simulink model "MotorControl_Bldc"  (R2022a)
settings: Solver=ode4  StartTime=0.0  StopTime=1  FixedStep=Ts/cnt_pTs  RelTol=1e-3
values from neighbouring files (symbols this model uses):
  cnt_pTs = 1000    [motorpara.m]
  Fc = 1/Ts    (= 10000)    [motorpara.m]
  Ki_id = Rs*Fc    (= 4500)    [motorpara.m]
  Ki_iq = Rs*Fc    (= 4500)    [motorpara.m]
  Ki_v = 0.93    [motorpara.m]
  Kp_id = Ls*Fc    (= 4.2)    [motorpara.m]
  Kp_iq = Ls*Fc    (= 4.2)    [motorpara.m]
  Kp_v = 0.05    [motorpara.m]
  Ls = 0.00042    [motorpara.m]
  P = 2    [motorpara.m]
  Rs = 0.45    [motorpara.m]
  SMO_Kslide = 10    [motorpara.m]
  Ts = 1/10000    (= 0.0001)    [motorpara.m]
  V = 12    [motorpara.m]
undefined symbols (not defined in the file or in its folder): DiscIntNeverNeededParam, sigbuilder_block
libraries: nesl_utility x83, fl_lib x67, ee_lib x49, simulink x13, slpidlib x3, mcbplantlib x2, autolibpmsmexterior x1
(part 4 of 4)

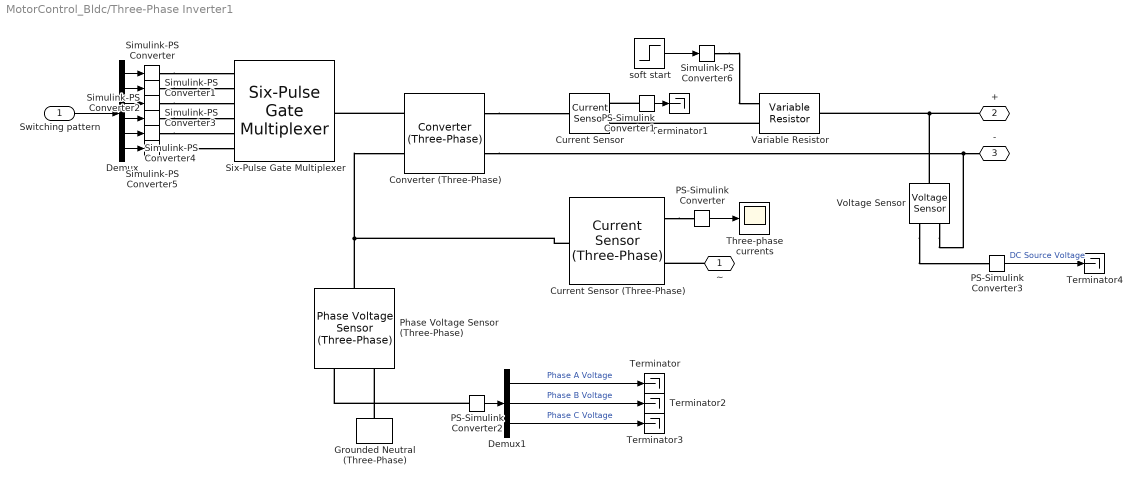
== system MotorControl_Bldc/Three-Phase Inverter1 ==
  Switching pattern : Inport
  Converter (Three-Phase) : ee_lib/Semiconductors & Converters/Converters/Converter (Three-Phase)  port_option=ee.enum.threePhasePort.composite  device_type=ee.enum.converters.switchingdevice.ideal  Vf=0.8 V  Ron=0.001 Ohm  Rds=0.001 Ohm  Goff=0.001 1/Ohm  Vgt=1 V  Vgt_off=-1 V  Ih=1 A  Vth=0.5 V  diode_param=ee.enum.converters.protectiondiode.nodynamics  diode_Vf=0.8 V  diode_Ron=0.001 Ohm  diode_Goff=1e-5 1/Ohm  diode_C=50 nF  diode_iRM=-235 A  diode_iF=300 A  diode_idot=-50 A/us  diode_trr_param=ee.enum.converters.diodetrr.trr_factor  diode_trr_factor=3  diode_trr=15 us  diode_Qrr=1500 s*uA  snubber_type=ee.enum.converters.snubber.exclude  Cs=1e-7 F  Rs=0.1 Ohm
      settings: SourceProductBaseCode=PS
  Current Sensor : fl_lib/Electrical/Electrical Sensors/Current Sensor
  Current Sensor (Three-Phase) : ee_lib/Sensors & Transducers/Current Sensor (Three-Phase)
  Demux : Demux  Outputs=6
  Demux1 : Demux  Outputs=3
  Grounded Neutral (Three-Phase) : ee_lib/Connectors & References/Grounded Neutral (Three-Phase)
      settings: SourceProductBaseCode=PS
  PS-Simulink Converter : nesl_utility/PS-Simulink Converter  PhysicalDomain=network_engine_domain  SubClassName=ps_output  LeftPortType=input  RightPortType=output  PseudoPeriodic=off  Frequencies=[]  VectorFormat=1-D array  Unit=1  AffineConversion=off
  PS-Simulink Converter1 : nesl_utility/PS-Simulink Converter  PhysicalDomain=network_engine_domain  SubClassName=ps_output  LeftPortType=input  RightPortType=output  PseudoPeriodic=off  Frequencies=[]  VectorFormat=1-D array  Unit=inherit  AffineConversion=off
  PS-Simulink Converter2 : nesl_utility/PS-Simulink Converter  PhysicalDomain=network_engine_domain  SubClassName=ps_output  LeftPortType=input  RightPortType=output  PseudoPeriodic=off  Frequencies=[]  VectorFormat=1-D array  Unit=inherit  AffineConversion=off
  PS-Simulink Converter3 : nesl_utility/PS-Simulink Converter  PhysicalDomain=network_engine_domain  SubClassName=ps_output  LeftPortType=input  RightPortType=output  PseudoPeriodic=off  Frequencies=[]  VectorFormat=1-D array  Unit=inherit  AffineConversion=off
  Phase Voltage Sensor (Three-Phase) : ee_lib/Sensors & Transducers/Phase Voltage Sensor (Three-Phase)
      settings: SourceProductBaseCode=PS
  Simulink-PS Converter{,1..6} (7 alike) : nesl_utility/Simulink-PS Converter  PhysicalDomain=network_engine_domain  SubClassName=ps_input  LeftPortType=input  RightPortType=output  PseudoPeriodic=off  Frequencies=[]  NoiseDistribution=none  NoiseParameters=[]  Unit=1  AffineConversion=off  FilteringAndDerivatives=provide  SimscapeFilterOrder=1  InputFilterTimeConstant=0.001  UdotUserProvided=0
  Six-Pulse Gate Multiplexer : ee_lib/Semiconductors & Converters/Converters/Six-Pulse Gate Multiplexer  port_option=ee.enum.controlport.ps
      settings: SourceProductBaseCode=PS
  Terminator{,1..4} (5 alike) : Terminator
  Three-phase currents : Scope
  Variable Resistor : fl_lib/Electrical/Electrical Elements/Variable Resistor  Rmin=0 Ohm  i_specify=off  i_priority=None  i=0 A  i_nominal_specify=off  i_nominal_unit=A  i_nominal_value=1  v_specify=off  v_priority=None  v=0 V  v_nominal_specify=off  v_nominal_unit=V  v_nominal_value=1
  Voltage Sensor : fl_lib/Electrical/Electrical Sensors/Voltage Sensor
  soft start : Step  Time=4  Before=0.5  After=1e-3  SampleTime=Ts
  ~ : PMIOPort  Side=Right
  + : PMIOPort  Port=2  Side=Left
  - : PMIOPort  Port=3  Side=Left
  wires:
  PS-Simulink Converter/1 -> Three-phase currents/1
  Switching pattern/1 -> Demux/1
  Demux/1 -> Simulink-PS Converter/1
  Demux/2 -> Simulink-PS Converter1/1
  Demux/3 -> Simulink-PS Converter2/1
  Demux/4 -> Simulink-PS Converter3/1
  Demux/5 -> Simulink-PS Converter4/1
  Demux/6 -> Simulink-PS Converter5/1
  PS-Simulink Converter2/1 -> Demux1/1
  soft start/1 -> Simulink-PS Converter6/1
  PS-Simulink Converter1/1 -> Terminator1/1
  Demux1/1 -> Terminator/1  "Phase A Voltage"
  Demux1/2 -> Terminator2/1  "Phase B Voltage"
  Demux1/3 -> Terminator3/1  "Phase C Voltage"
  PS-Simulink Converter3/1 -> Terminator4/1  "DC Source Voltage"
  connections:
  Current Sensor (Three-Phase)/RConn1 -- PS-Simulink Converter/LConn1
  Simulink-PS Converter/RConn1 -- Six-Pulse Gate Multiplexer/LConn1
  Simulink-PS Converter1/RConn1 -- Six-Pulse Gate Multiplexer/LConn2
  Simulink-PS Converter2/RConn1 -- Six-Pulse Gate Multiplexer/LConn3
  Simulink-PS Converter3/RConn1 -- Six-Pulse Gate Multiplexer/LConn4
  Simulink-PS Converter4/RConn1 -- Six-Pulse Gate Multiplexer/LConn5
  Simulink-PS Converter5/RConn1 -- Six-Pulse Gate Multiplexer/LConn6
  Converter (Three-Phase)/LConn1 -- Six-Pulse Gate Multiplexer/RConn1
  Converter (Three-Phase)/RConn1 -- Current Sensor/LConn1
  Converter (Three-Phase)/RConn2 -- Voltage Sensor/RConn2 -- -/RConn1
  Current Sensor (Three-Phase)/LConn1 -- Converter (Three-Phase)/LConn2 -- Phase Voltage Sensor (Three-Phase)/LConn1
  ~/RConn1 -- Current Sensor (Three-Phase)/RConn2
  Grounded Neutral (Three-Phase)/LConn1 -- Phase Voltage Sensor (Three-Phase)/RConn2
  PS-Simulink Converter2/LConn1 -- Phase Voltage Sensor (Three-Phase)/RConn1
  PS-Simulink Converter1/LConn1 -- Current Sensor/RConn1
  Variable Resistor/LConn2 -- Current Sensor/RConn2
  +/RConn1 -- Voltage Sensor/LConn1 -- Variable Resistor/RConn1
  Simulink-PS Converter6/RConn1 -- Variable Resistor/LConn1
  Voltage Sensor/RConn1 -- PS-Simulink Converter3/LConn1

== system MotorControl_Bldc/Tload1 ==
  Simulink-PS Converter4 : nesl_utility/Simulink-PS Converter  PhysicalDomain=network_engine_domain  SubClassName=ps_input  LeftPortType=input  RightPortType=output  PseudoPeriodic=off  Frequencies=[]  NoiseDistribution=none  NoiseParameters=[]  Unit=N*m  AffineConversion=off  FilteringAndDerivatives=zero  SimscapeFilterOrder=1  InputFilterTimeConstant=0.001  UdotUserProvided=1
      settings: SourceProductBaseCode=SS,PW,VE
  Step : Step  Time=0.9  After=-2  SampleTime=0
  Tload : PMIOPort  Side=Right
  wires:
  Step/1 -> Simulink-PS Converter4/1
  connections:
  Simulink-PS Converter4/RConn1 -- Tload/RConn1

== system MotorControl_Bldc/Tload3 ==
  Simulink-PS Converter4 : nesl_utility/Simulink-PS Converter  PhysicalDomain=network_engine_domain  SubClassName=ps_input  LeftPortType=input  RightPortType=output  PseudoPeriodic=off  Frequencies=[]  NoiseDistribution=none  NoiseParameters=[]  Unit=N*m  AffineConversion=off  FilteringAndDerivatives=zero  SimscapeFilterOrder=1  InputFilterTimeConstant=0.001  UdotUserProvided=1
      settings: SourceProductBaseCode=SS,PW,VE
  Step : Step  Time=0.9  After=-2  SampleTime=0
  Tload : PMIOPort  Side=Right
  wires:
  Step/1 -> Simulink-PS Converter4/1
  connections:
  Simulink-PS Converter4/RConn1 -- Tload/RConn1

== system MotorControl_Bldc/clark ==
  PhI : Inport
  Add : Sum
  Demux : Demux  Outputs=3
  Gain : Gain  Gain=2
  Gain1 : Gain  Gain=1/sqrt(3)
  Scope : Scope
  Iα : Outport
  Iβ : Outport  Port=2
  wires:
  PhI/1 -> Demux/1
  Demux/1 -> Add/1, Iα/1
  Demux/2 -> Gain/1
  Gain/1 -> Add/2
  Add/1 -> Gain1/1
  Gain1/1 -> Iβ/1
  Demux/3 -> Scope/1

== system MotorControl_Bldc/ref_ratio ==
  alpha : Inport
  lead : Inport  Port=2
  leg : Inport  Port=3
  Add7 : Sum
  Cos : Trigonometry  Operator=cos
  Sin : Trigonometry
  Sqrt : Sqrt
  ap : Product
  bp : Product
  mcos : Product
  msin : Product
  module : Outport
  wires:
  ap/1 -> msin/2, msin/1
  Add7/1 -> Sqrt/1
  Cos/1 -> bp/1
  mcos/1 -> Add7/2
  Sin/1 -> ap/2
  alpha/1 -> Cos/1, Sin/1
  bp/1 -> mcos/1, mcos/2
  Sqrt/1 -> module/1
  msin/1 -> Add7/1
  lead/1 -> bp/2
  leg/1 -> ap/1

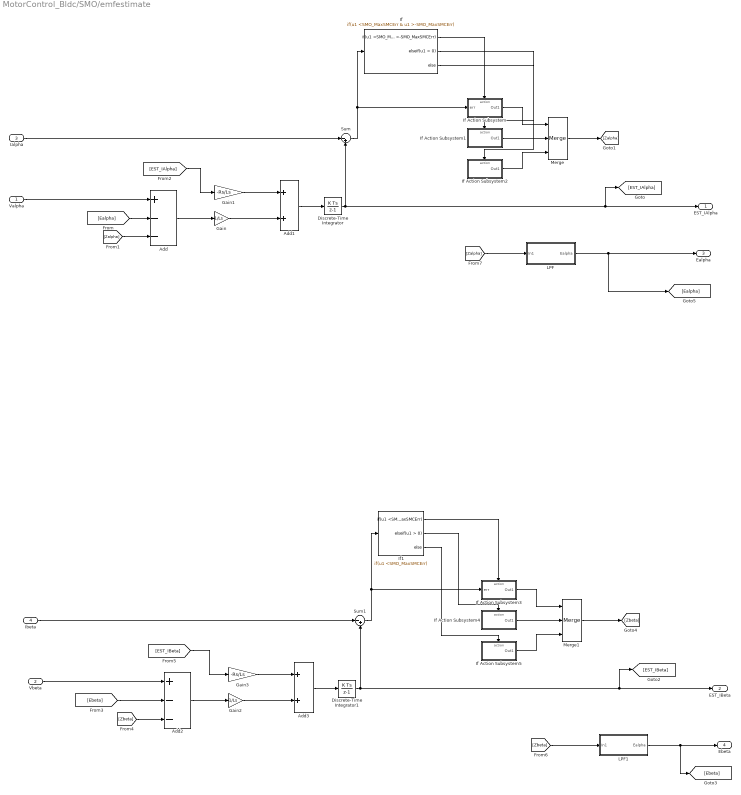
== system MotorControl_Bldc/SMO/emfestimate ==
  Valpha : Inport
  Vbeta : Inport  Port=2
  Ialpha : Inport  Port=3
  Ibeta : Inport  Port=4
  Add : Sum  Inputs=+--
  Add1 : Sum
  Add2 : Sum  Inputs=+--
  Add3 : Sum
  Discrete-Time Integrator : DiscreteIntegrator  SampleTime=Ts  ICPrevOutput=DiscIntNeverNeededParam  ICPrevScaledInput=DiscIntNeverNeededParam
  Discrete-Time Integrator1 : DiscreteIntegrator  SampleTime=Ts  ICPrevOutput=DiscIntNeverNeededParam  ICPrevScaledInput=DiscIntNeverNeededParam
  Gain : Gain  Gain=1/Ls
  Gain1 : Gain  Gain=-Rs/Ls
  Gain2 : Gain  Gain=1/Ls
  Gain3 : Gain  Gain=-Rs/Ls
  If : If  IfExpression=u1 <SMO_MaxSMCErr & u1 >-SMO_MaxSMCErr  ElseIfExpressions=u1 > 0
  If Action Subsystem : Subsystem  TreatAsAtomicUnit=on
  If Action Subsystem1 : Subsystem  TreatAsAtomicUnit=on
  If Action Subsystem2 : Subsystem  TreatAsAtomicUnit=on
  If Action Subsystem3 : Subsystem  TreatAsAtomicUnit=on
  If Action Subsystem4 : Subsystem  TreatAsAtomicUnit=on
  If Action Subsystem5 : Subsystem  TreatAsAtomicUnit=on
  If1 : If  IfExpression=u1 <SMO_MaxSMCErr  ElseIfExpressions=u1 > 0
  LPF : Subsystem
  LPF1 : Subsystem
  Merge : Merge  Inputs=3
  Merge1 : Merge  Inputs=3
  Sum : Sum  Inputs=|-+
  Sum1 : Sum  Inputs=|-+
  EST_IAlpha : Outport
  EST_IBeta : Outport  Port=2
  Ealpha : Outport  Port=3
  Ebeta : Outport  Port=4
  wires:
  Valpha/1 -> Add/1
  Add/1 -> Gain/1
  [Ealpha] -> Add/2
  [Zalpha] -> Add/3
  Gain/1 -> Add1/2
  Gain1/1 -> Add1/1
  [EST_IAlpha] -> Gain1/1
  Add1/1 -> Discrete-Time Integrator/1
  Discrete-Time Integrator/1 -> [EST_IAlpha], EST_IAlpha/1, Sum/2
  Ialpha/1 -> Sum/1
  Sum/1 -> If/1, If Action Subsystem/1(err)
  If/1 -> If Action Subsystem/Action
  If/2 -> If Action Subsystem1/Action
  If/3 -> If Action Subsystem2/Action
  If Action Subsystem1/1(Out1) -> Merge/2
  If Action Subsystem/1(Out1) -> Merge/1
  If Action Subsystem2/1(Out1) -> Merge/3
  Merge/1 -> [Zalpha]
  Add3/1 -> Discrete-Time Integrator1/1
  [Zbeta] -> Add2/3
  If Action Subsystem5/1(Out1) -> Merge1/3
  Gain2/1 -> Add3/2
  Merge1/1 -> [Zbeta]
  If Action Subsystem3/1(Out1) -> Merge1/1
  If Action Subsystem4/1(Out1) -> Merge1/2
  Vbeta/1 -> Add2/1
  [Ebeta] -> Add2/2
  Ibeta/1 -> Sum1/1
  Sum1/1 -> If1/1, If Action Subsystem3/1(err)
  If1/3 -> If Action Subsystem5/Action
  If1/1 -> If Action Subsystem3/Action
  Gain3/1 -> Add3/1
  Discrete-Time Integrator1/1 -> EST_IBeta/1, [EST_IBeta], Sum1/2
  [EST_IBeta] -> Gain3/1
  If1/2 -> If Action Subsystem4/Action
  Add2/1 -> Gain2/1
  LPF/1(Ealpha) -> [Ealpha], Ealpha/1
  [Zalpha] -> LPF/1(In1)
  LPF1/1(Ealpha) -> [Ebeta], Ebeta/1
  [Zbeta] -> LPF1/1(In1)

== system MotorControl_Bldc/SMO/vmeasure ==
  last : Inport
  this : Inport  Port=2
  Add : Sum  Inputs=-+
  Constant : Constant  Value=Ts
  Divide : Product  Inputs=*/
  Gain : Gain  Gain=30/pi
  If : If  IfExpression=u1 > 4.7  ElseIfExpressions=u1<-4.7
  If Action Subsystem : Subsystem  TreatAsAtomicUnit=on
  If Action Subsystem1 : Subsystem  TreatAsAtomicUnit=on
  If Action Subsystem2 : Subsystem  TreatAsAtomicUnit=on
  Merge : Merge  Inputs=3
  Saturation : Saturate  UpperLimit=5000  LowerLimit=-5000
  Out1 : Outport
  wires:
  last/1 -> If Action Subsystem/2(last), If Action Subsystem1/2(last), Add/1
  this/1 -> If Action Subsystem1/1(this), If Action Subsystem/1(this), Add/2
  Add/1 -> If/1, If Action Subsystem2/1(In1)
  If/1 -> If Action Subsystem/Action
  If/2 -> If Action Subsystem1/Action
  If/3 -> If Action Subsystem2/Action
  If Action Subsystem2/1(Out1) -> Merge/2
  If Action Subsystem/1(Out1) -> Merge/1
  Merge/1 -> Divide/1
  Divide/1 -> Gain/1
  Constant/1 -> Divide/2
  If Action Subsystem1/1(Out1) -> Merge/3
  Gain/1 -> Saturation/1
  Saturation/1 -> Out1/1

== system MotorControl_Bldc/SVPWM/Sector ==
  Vα : Inport
  Vβ : Inport  Port=2
  Add : Sum  Inputs=+-
  Add1 : Sum  Inputs=--
  Add2 : Sum  Inputs=+++
  Constant : Constant
  Constant1 : Constant  Value=0
  Gain : Gain  Gain=sqrt(3)
  Gain1 : Gain  Gain=4
  Gain2 : Gain  Gain=2
  Gain3 : Gain
  Switch : Switch  Criteria=u2 > Threshold  SaturateOnIntegerOverflow=off  InputSameDT=off
  Switch1 : Switch  Criteria=u2 > Threshold  SaturateOnIntegerOverflow=off  InputSameDT=off
  Switch2 : Switch  Criteria=u2 > Threshold  SaturateOnIntegerOverflow=off  InputSameDT=off
  N : Outport
  wires:
  Vα/1 -> Gain/1
  Gain/1 -> Add1/1, Add/1
  Vβ/1 -> Add1/2, Switch/2, Add/2
  Add/1 -> Switch1/2
  Add1/1 -> Switch2/2
  Constant1/1 -> Switch/3, Switch1/3, Switch2/3
  Constant/1 -> Switch2/1, Switch1/1, Switch/1
  Switch/1 -> Gain3/1
  Switch1/1 -> Gain2/1
  Switch2/1 -> Gain1/1
  Gain3/1 -> Add2/1
  Gain2/1 -> Add2/2
  Gain1/1 -> Add2/3
  Add2/1 -> N/1

== system MotorControl_Bldc/SVPWM/Subsystem ==
  N : Inport
  T1 : Inport  Port=2
  T2 : Inport  Port=3
  TS : Inport  Port=4
  Add : Sum  Inputs=--+
  Gain : Gain  Gain=0.5
  Gain1 : Gain  Gain=0.5
  Gain2 : Gain  Gain=1/4
  Index Vector : MultiPortSwitch  Inputs=6  DiagnosticForDefault=None  SaturateOnIntegerOverflow=off  InputSameDT=off
  Index Vector1 : MultiPortSwitch  Inputs=6  DiagnosticForDefault=None  SaturateOnIntegerOverflow=off  InputSameDT=off
  Index Vector2 : MultiPortSwitch  Inputs=6  DiagnosticForDefault=None  SaturateOnIntegerOverflow=off  InputSameDT=off
  mid1 : Sum
  mid2 : Sum
  Ta : Outport
  Tb : Outport  Port=2
  Tc : Outport  Port=3
  wires:
  T1/1 -> Add/2, Gain1/1
  T2/1 -> Add/1, Gain/1
  TS/1 -> Add/3
  Add/1 -> Gain2/1
  Gain/1 -> mid1/1
  Gain1/1 -> mid2/1
  mid2/1 -> Index Vector2/6, Index Vector2/3, Index Vector1/5, Index Vector1/4, Index Vector/7, Index Vector/2, mid1/2
  Gain2/1 -> Index Vector1/6, Index Vector1/2, Index Vector/4, Index Vector/3, mid2/2, Index Vector2/7, Index Vector2/5
  N/1 -> Index Vector2/1, Index Vector1/1, Index Vector/1
  mid1/1 -> Index Vector/6, Index Vector/5, Index Vector1/7, Index Vector2/4, Index Vector2/2, Index Vector1/3
  Index Vector/1 -> Ta/1
  Index Vector1/1 -> Tb/1
  Index Vector2/1 -> Tc/1

== system MotorControl_Bldc/SVPWM/T1T2 ==
  N : Inport
  X : Inport  Port=2
  Y : Inport  Port=3
  Z : Inport  Port=4
  Gain : Gain  Gain=-1
  Gain1 : Gain  Gain=-1
  Gain2 : Gain  Gain=-1
  Index Vector : MultiPortSwitch  Inputs=6  DiagnosticForDefault=None  SaturateOnIntegerOverflow=off  InputSameDT=off
  Index Vector1 : MultiPortSwitch  Inputs=6  DiagnosticForDefault=None  SaturateOnIntegerOverflow=off  InputSameDT=off
  T1 : Outport
  T2 : Outport  Port=2
  wires:
  X/1 -> Gain/1, Index Vector/6, Index Vector1/4
  Index Vector1/1 -> T2/1
  N/1 -> Index Vector1/1, Index Vector/1
  Y/1 -> Gain1/1, Index Vector/3, Index Vector1/2
  Z/1 -> Gain2/1, Index Vector1/5, Index Vector/2
  Gain/1 -> Index Vector1/3, Index Vector/5
  Gain2/1 -> Index Vector1/7, Index Vector/4
  Gain1/1 -> Index Vector/7, Index Vector1/6
  Index Vector/1 -> T1/1

== system MotorControl_Bldc/SVPWM/XYZ ==
  Vα : Inport
  Vβ : Inport  Port=2
  Vbus : Inport  Port=3
  TS : Inport  Port=4
  Add : Sum  Inputs=+-
  Add1 : Sum  Inputs=--
  Constant : Constant  Value=sqrt(3)
  Divide : Product  Inputs=**/
  Gain : Gain  Gain=sqrt(3)
  Gain1 : Gain  Gain=-0.5
  Gain2 : Gain  Gain=-0.5
  Product : Product
  Product1 : Product
  Product2 : Product
  X : Outport
  Y : Outport  Port=2
  Z : Outport  Port=3
  wires:
  Vα/1 -> Gain/1
  Gain/1 -> Add/1, Add1/1
  Vβ/1 -> Add1/2, Product/1, Add/2
  Add1/1 -> Gain1/1
  Add/1 -> Gain2/1
  Constant/1 -> Divide/1
  Vbus/1 -> Divide/3
  TS/1 -> Divide/2
  Gain1/1 -> Product1/1
  Divide/1 -> Product2/2, Product/2, Product1/2
  Product2/1 -> Z/1
  Product1/1 -> Y/1
  Product/1 -> X/1
  Gain2/1 -> Product2/1

== system MotorControl_Bldc/SVPWM1/Sector ==
  Vα : Inport
  Vβ : Inport  Port=2
  Add : Sum  Inputs=+-
  Add1 : Sum  Inputs=--
  Add2 : Sum  Inputs=+++
  Constant : Constant
  Constant1 : Constant  Value=0
  Gain : Gain  Gain=sqrt(3)
  Gain1 : Gain  Gain=4
  Gain2 : Gain  Gain=2
  Gain3 : Gain
  Switch : Switch  Criteria=u2 > Threshold  SaturateOnIntegerOverflow=off  InputSameDT=off
  Switch1 : Switch  Criteria=u2 > Threshold  SaturateOnIntegerOverflow=off  InputSameDT=off
  Switch2 : Switch  Criteria=u2 > Threshold  SaturateOnIntegerOverflow=off  InputSameDT=off
  N : Outport
  wires:
  Vα/1 -> Gain/1
  Gain/1 -> Add1/1, Add/1
  Vβ/1 -> Add1/2, Switch/2, Add/2
  Add/1 -> Switch1/2
  Add1/1 -> Switch2/2
  Constant1/1 -> Switch/3, Switch1/3, Switch2/3
  Constant/1 -> Switch2/1, Switch1/1, Switch/1
  Switch/1 -> Gain3/1
  Switch1/1 -> Gain2/1
  Switch2/1 -> Gain1/1
  Gain3/1 -> Add2/1
  Gain2/1 -> Add2/2
  Gain1/1 -> Add2/3
  Add2/1 -> N/1

== system MotorControl_Bldc/SVPWM1/Subsystem ==
  N : Inport
  T1 : Inport  Port=2
  T2 : Inport  Port=3
  TS : Inport  Port=4
  Add : Sum  Inputs=--+
  Gain : Gain  Gain=0.5
  Gain1 : Gain  Gain=0.5
  Gain2 : Gain  Gain=1/4
  Index Vector : MultiPortSwitch  Inputs=6  DiagnosticForDefault=None  SaturateOnIntegerOverflow=off  InputSameDT=off
  Index Vector1 : MultiPortSwitch  Inputs=6  DiagnosticForDefault=None  SaturateOnIntegerOverflow=off  InputSameDT=off
  Index Vector2 : MultiPortSwitch  Inputs=6  DiagnosticForDefault=None  SaturateOnIntegerOverflow=off  InputSameDT=off
  mid1 : Sum
  mid2 : Sum
  Ta : Outport
  Tb : Outport  Port=2
  Tc : Outport  Port=3
  wires:
  T1/1 -> Add/2, Gain1/1
  T2/1 -> Add/1, Gain/1
  TS/1 -> Add/3
  Add/1 -> Gain2/1
  Gain/1 -> mid1/1
  Gain1/1 -> mid2/1
  mid2/1 -> Index Vector2/6, Index Vector2/3, Index Vector1/5, Index Vector1/4, Index Vector/7, Index Vector/2, mid1/2
  Gain2/1 -> Index Vector1/6, Index Vector1/2, Index Vector/4, Index Vector/3, mid2/2, Index Vector2/7, Index Vector2/5
  N/1 -> Index Vector2/1, Index Vector1/1, Index Vector/1
  mid1/1 -> Index Vector/6, Index Vector/5, Index Vector1/7, Index Vector2/4, Index Vector2/2, Index Vector1/3
  Index Vector/1 -> Ta/1
  Index Vector1/1 -> Tb/1
  Index Vector2/1 -> Tc/1

== system MotorControl_Bldc/SVPWM1/T1T2 ==
  N : Inport
  X : Inport  Port=2
  Y : Inport  Port=3
  Z : Inport  Port=4
  Gain : Gain  Gain=-1
  Gain1 : Gain  Gain=-1
  Gain2 : Gain  Gain=-1
  Index Vector : MultiPortSwitch  Inputs=6  DiagnosticForDefault=None  SaturateOnIntegerOverflow=off  InputSameDT=off
  Index Vector1 : MultiPortSwitch  Inputs=6  DiagnosticForDefault=None  SaturateOnIntegerOverflow=off  InputSameDT=off
  T1 : Outport
  T2 : Outport  Port=2
  wires:
  X/1 -> Gain/1, Index Vector/6, Index Vector1/4
  Index Vector1/1 -> T2/1
  N/1 -> Index Vector1/1, Index Vector/1
  Y/1 -> Gain1/1, Index Vector/3, Index Vector1/2
  Z/1 -> Gain2/1, Index Vector1/5, Index Vector/2
  Gain/1 -> Index Vector1/3, Index Vector/5
  Gain2/1 -> Index Vector1/7, Index Vector/4
  Gain1/1 -> Index Vector/7, Index Vector1/6
  Index Vector/1 -> T1/1

== system MotorControl_Bldc/SVPWM1/XYZ ==
  Vα : Inport
  Vβ : Inport  Port=2
  Vbus : Inport  Port=3
  TS : Inport  Port=4
  Add : Sum  Inputs=+-
  Add1 : Sum  Inputs=--
  Constant : Constant  Value=sqrt(3)
  Divide : Product  Inputs=**/
  Gain : Gain  Gain=sqrt(3)
  Gain1 : Gain  Gain=-0.5
  Gain2 : Gain  Gain=-0.5
  Product : Product
  Product1 : Product
  Product2 : Product
  X : Outport
  Y : Outport  Port=2
  Z : Outport  Port=3
  wires:
  Vα/1 -> Gain/1
  Gain/1 -> Add/1, Add1/1
  Vβ/1 -> Add1/2, Product/1, Add/2
  Add1/1 -> Gain1/1
  Add/1 -> Gain2/1
  Constant/1 -> Divide/1
  Vbus/1 -> Divide/3
  TS/1 -> Divide/2
  Gain1/1 -> Product1/1
  Divide/1 -> Product2/2, Product/2, Product1/2
  Product2/1 -> Z/1
  Product1/1 -> Y/1
  Product/1 -> X/1
  Gain2/1 -> Product2/1

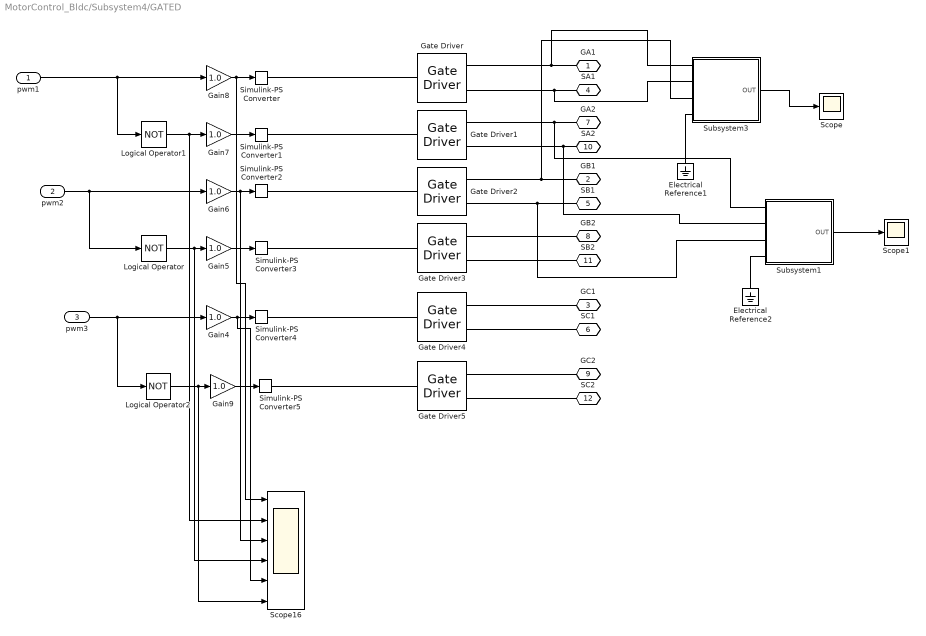
== system MotorControl_Bldc/Subsystem4/GATED ==
  pwm1 : Inport
  pwm2 : Inport  Port=2
  pwm3 : Inport  Port=3
  Electrical Reference1 : fl_lib/Electrical/Electrical Elements/Electrical Reference
      settings: SourceProductBaseCode=PW,SS,VE
  Electrical Reference2 : fl_lib/Electrical/Electrical Elements/Electrical Reference
      settings: SourceProductBaseCode=PW,SS,VE
  Gain{4..9} (6 alike) : Gain  Gain=1.0  OutDataTypeStr=double
  Gate Driver{,1..5} (6 alike) : ee_lib/Semiconductors & Converters/Gate Driver  uHighValue=0.7  uLowValue=0.3  vHigh=15 V  vLow=0 V  tHigh=50 ns  tLow=50 ns  parameterization=1  rHigh=2 Ohm  rLow=2 Ohm  tRise=20 ns  tFall=20 ns  cLoad=10 nF  enable_faults=0  t_fault=1 s  fault_type=1  ZonTime_specify=off  ZonTime_priority=None  ZonTime=0 s  ZoffTime_specify=off  ZoffTime_priority=None  ZoffTime=0 s  uHigh=2.0 V  uLow=0.8 V
      settings: SourceProductBaseCode=PS  InternalSimscapePortConfiguration="{\"Bottom\":[],\"Left\":[{\"id\":\"u\",\"label\":\"u\",\"type\":\"input\"}],\"Right\":[{\"id\":\"G\",\"label\":\"G\",\"type\":\"foundation.electrical.electrical\"},{\"id\":\"S\",\"label\":\"S\",\"type\":\"foundation.electrical.electrical\"}],\"Top\":[]}"
  Logical Operator : Logic  Operator=NOT  AllPortsSameDT=off  OutDataTypeStr=boolean
  Logical Operator1 : Logic  Operator=NOT  AllPortsSameDT=off  OutDataTypeStr=boolean
  Logical Operator2 : Logic  Operator=NOT  AllPortsSameDT=off  OutDataTypeStr=boolean
  Scope : Scope
  Scope1 : Scope
  Scope16 : Scope  NumInputPorts=6
  Simulink-PS Converter{,1..5} (6 alike) : nesl_utility/Simulink-PS Converter  PhysicalDomain=network_engine_domain  SubClassName=ps_input  LeftPortType=input  RightPortType=output  PseudoPeriodic=off  Frequencies=[]  NoiseDistribution=none  NoiseParameters=[]  Unit=1  AffineConversion=off  FilteringAndDerivatives=provide  SimscapeFilterOrder=1  InputFilterTimeConstant=0.001  UdotUserProvided=0
      settings: SourceProductBaseCode=SS,PW,VE
  Subsystem1 : Subsystem
  Subsystem3 : Subsystem
  GA1 : PMIOPort  Side=Right
  GB1 : PMIOPort  Port=2  Side=Right
  GC1 : PMIOPort  Port=3  Side=Right
  SA1 : PMIOPort  Port=4  Side=Right
  SB1 : PMIOPort  Port=5  Side=Right
  SC1 : PMIOPort  Port=6  Side=Right
  GA2 : PMIOPort  Port=7  Side=Right
  GB2 : PMIOPort  Port=8  Side=Right
  GC2 : PMIOPort  Port=9  Side=Right
  SA2 : PMIOPort  Port=10  Side=Right
  SB2 : PMIOPort  Port=11  Side=Right
  SC2 : PMIOPort  Port=12  Side=Right
  wires:
  Logical Operator2/1 -> Scope16/6, Gain9/1
  pwm2/1 -> Gain6/1, Logical Operator/1
  Gain5/1 -> Simulink-PS Converter3/1
  pwm3/1 -> Gain4/1, Logical Operator2/1
  Gain4/1 -> Scope16/5, Simulink-PS Converter4/1
  pwm1/1 -> Gain8/1, Logical Operator1/1
  Logical Operator/1 -> Scope16/4, Gain5/1
  Gain6/1 -> Scope16/3, Simulink-PS Converter2/1
  Gain7/1 -> Simulink-PS Converter1/1
  Gain8/1 -> Scope16/1, Simulink-PS Converter/1
  Gain9/1 -> Simulink-PS Converter5/1
  Logical Operator1/1 -> Scope16/2, Gain7/1
  Subsystem3/1(OUT) -> Scope/1
  Subsystem1/1(OUT) -> Scope1/1
  connections:
  Gate Driver3/LConn1 -- Simulink-PS Converter3/RConn1
  Gate Driver5/LConn1 -- Simulink-PS Converter5/RConn1
  Gate Driver/LConn1 -- Simulink-PS Converter/RConn1
  Gate Driver1/LConn1 -- Simulink-PS Converter1/RConn1
  Simulink-PS Converter2/RConn1 -- Gate Driver2/LConn1
  Gate Driver4/LConn1 -- Simulink-PS Converter4/RConn1
  GA1/RConn1 -- Subsystem3/LConn1 -- Gate Driver/RConn1
  SA1/RConn1 -- Subsystem3/LConn2 -- Gate Driver/RConn2
  GA2/RConn1 -- Subsystem1/LConn1 -- Gate Driver1/RConn1
  SA2/RConn1 -- Subsystem1/LConn2 -- Gate Driver1/RConn2
  GB1/RConn1 -- Subsystem3/LConn3 -- Gate Driver2/RConn1
  SB1/RConn1 -- Subsystem1/LConn3 -- Gate Driver2/RConn2
  GB2/RConn1 -- Gate Driver3/RConn1
  SB2/RConn1 -- Gate Driver3/RConn2
  GC1/RConn1 -- Gate Driver4/RConn1
  SC1/RConn1 -- Gate Driver4/RConn2
  GC2/RConn1 -- Gate Driver5/RConn1
  SC2/RConn1 -- Gate Driver5/RConn2
  Electrical Reference1/LConn1 -- Subsystem3/LConn4
  Electrical Reference2/LConn1 -- Subsystem1/LConn4

== system MotorControl_Bldc/Subsystem4/Subsystem3 ==
  Mux4 : Mux  Inputs=3
  PS-Simulink Converter : nesl_utility/PS-Simulink Converter  PhysicalDomain=network_engine_domain  SubClassName=ps_output  LeftPortType=input  RightPortType=output  PseudoPeriodic=off  Frequencies=[]  VectorFormat=inherit  Unit=inherit  AffineConversion=off
      settings: SourceProductBaseCode=SS,PW,VE
  PS-Simulink Converter1 : nesl_utility/PS-Simulink Converter  PhysicalDomain=network_engine_domain  SubClassName=ps_output  LeftPortType=input  RightPortType=output  PseudoPeriodic=off  Frequencies=[]  VectorFormat=1-D array  Unit=V  AffineConversion=off
      settings: SourceProductBaseCode=SS,PW,VE
  PS-Simulink Converter2 : nesl_utility/PS-Simulink Converter  PhysicalDomain=network_engine_domain  SubClassName=ps_output  LeftPortType=input  RightPortType=output  PseudoPeriodic=off  Frequencies=[]  VectorFormat=1-D array  Unit=V  AffineConversion=off
      settings: SourceProductBaseCode=SS,PW,VE
  Voltage Sensor1 : fl_lib/Electrical/Electrical Sensors/Voltage Sensor
      settings: SourceProductBaseCode=PW,SS,VE
  Voltage Sensor2 : fl_lib/Electrical/Electrical Sensors/Voltage Sensor
      settings: SourceProductBaseCode=PW,SS,VE
  Voltage Sensor3 : fl_lib/Electrical/Electrical Sensors/Voltage Sensor
      settings: SourceProductBaseCode=PW,SS,VE
  AV : PMIOPort  Port=2  Side=Left
  CV : PMIOPort  Port=3  Side=Left
  BV : PMIOPort  Port=4  Side=Left
  GND : PMIOPort  Port=5  Side=Left
  OUT : Outport
  wires:
  PS-Simulink Converter/1 -> Mux4/3
  PS-Simulink Converter1/1 -> Mux4/1
  PS-Simulink Converter2/1 -> Mux4/2
  Mux4/1 -> OUT/1
  connections:
  Voltage Sensor3/RConn2 -- Voltage Sensor1/RConn2 -- Voltage Sensor2/RConn2 -- GND/RConn1
  PS-Simulink Converter1/LConn1 -- Voltage Sensor1/RConn1
  Voltage Sensor3/LConn1 -- CV/RConn1
  PS-Simulink Converter2/LConn1 -- Voltage Sensor2/RConn1
  Voltage Sensor1/LConn1 -- AV/RConn1
  PS-Simulink Converter/LConn1 -- Voltage Sensor3/RConn1
  Voltage Sensor2/LConn1 -- BV/RConn1

== system MotorControl_Bldc/SMO/emfestimate/If Action Subsystem ==
  err : Inport
  Action Port : ActionPort  ActionPortLabel=if(u1 <SMO_MaxSMCErr & u1 >-SMO_MaxSMCErr)
  Constant : Constant  Value=SMO_Kslide
  Constant1 : Constant  Value=SMO_Kslide
  Divide : Product  Inputs=**
  Divide1 : Product  Inputs=*/
  Out1 : Outport
  wires:
  Constant/1 -> Divide/1
  err/1 -> Divide/2
  Divide/1 -> Divide1/1
  Divide1/1 -> Out1/1
  Constant1/1 -> Divide1/2

== system MotorControl_Bldc/SMO/emfestimate/If Action Subsystem1 ==
  Action Port : ActionPort  ActionPortLabel=elseif(u1 > 0)
  Constant : Constant  Value=SMO_Kslide
  Out1 : Outport
  wires:
  Constant/1 -> Out1/1

== system MotorControl_Bldc/SMO/emfestimate/If Action Subsystem2 ==
  Action Port : ActionPort  ActionPortLabel=else
  Constant : Constant  Value=SMO_Kslide
  Gain : Gain  Gain=-1
  Out1 : Outport
  wires:
  Constant/1 -> Gain/1
  Gain/1 -> Out1/1

== system MotorControl_Bldc/SMO/emfestimate/If Action Subsystem3 ==
  err : Inport
  Action Port : ActionPort  ActionPortLabel=if(u1 <SMO_MaxSMCErr)
  Constant : Constant  Value=SMO_Kslide
  Constant1 : Constant  Value=SMO_Kslide
  Divide : Product  Inputs=**
  Divide1 : Product  Inputs=*/
  Out1 : Outport
  wires:
  Constant/1 -> Divide/1
  err/1 -> Divide/2
  Divide/1 -> Divide1/1
  Divide1/1 -> Out1/1
  Constant1/1 -> Divide1/2

== system MotorControl_Bldc/SMO/emfestimate/If Action Subsystem4 ==
  Action Port : ActionPort  ActionPortLabel=elseif(u1 > 0)
  Constant : Constant  Value=SMO_Kslide
  Out1 : Outport
  wires:
  Constant/1 -> Out1/1

== system MotorControl_Bldc/SMO/emfestimate/If Action Subsystem5 ==
  Action Port : ActionPort  ActionPortLabel=else
  Constant : Constant  Value=SMO_Kslide
  Gain : Gain  Gain=-1
  Out1 : Outport
  wires:
  Constant/1 -> Gain/1
  Gain/1 -> Out1/1

== system MotorControl_Bldc/SMO/emfestimate/LPF ==
  In1 : Inport
  Add : Sum  Inputs=+-
  Add1 : Sum
  Constant : Constant  Value=0.05
  Divide : Product  Inputs=**
  Unit Delay : UnitDelay  SampleTime=-1  HasFrameUpgradeWarning=on
  Ealpha : Outport
  wires:
  In1/1 -> Add/1
  Constant/1 -> Divide/1
  Add/1 -> Divide/2
  Divide/1 -> Add1/1
  Add1/1 -> Unit Delay/1, Ealpha/1
  Unit Delay/1 -> Add1/2, Add/2

== system MotorControl_Bldc/SMO/emfestimate/LPF1 ==
  In1 : Inport
  Add : Sum  Inputs=+-
  Add1 : Sum
  Constant : Constant  Value=0.05
  Divide : Product  Inputs=**
  Unit Delay : UnitDelay  SampleTime=-1  HasFrameUpgradeWarning=on
  Ealpha : Outport
  wires:
  In1/1 -> Add/1
  Constant/1 -> Divide/1
  Add/1 -> Divide/2
  Divide/1 -> Add1/1
  Add1/1 -> Unit Delay/1, Ealpha/1
  Unit Delay/1 -> Add1/2, Add/2

== system MotorControl_Bldc/SMO/vmeasure/If Action Subsystem ==
  this : Inport
  last : Inport  Port=2
  Action Port : ActionPort  ActionPortLabel=if(u1 > 4.7)
  Add : Sum  Inputs=+--
  Constant : Constant  Value=2*pi
  Out1 : Outport
  wires:
  Constant/1 -> Add/2
  this/1 -> Add/1
  last/1 -> Add/3
  Add/1 -> Out1/1

== system MotorControl_Bldc/SMO/vmeasure/If Action Subsystem1 ==
  this : Inport
  last : Inport  Port=2
  Action Port : ActionPort  ActionPortLabel=elseif(u1<-4.7)
  Add : Sum  Inputs=++-
  Constant : Constant  Value=2*pi
  Out1 : Outport
  wires:
  Constant/1 -> Add/1
  this/1 -> Add/2
  last/1 -> Add/3
  Add/1 -> Out1/1

== system MotorControl_Bldc/SMO/vmeasure/If Action Subsystem2 ==
  In1 : Inport
  Action Port : ActionPort  ActionPortLabel=else
  Out1 : Outport
  wires:
  In1/1 -> Out1/1

== system MotorControl_Bldc/Subsystem4/GATED/Subsystem1 ==
  Mux4 : Mux  Inputs=3
  PS-Simulink Converter : nesl_utility/PS-Simulink Converter  PhysicalDomain=network_engine_domain  SubClassName=ps_output  LeftPortType=input  RightPortType=output  PseudoPeriodic=off  Frequencies=[]  VectorFormat=inherit  Unit=inherit  AffineConversion=off
      settings: SourceProductBaseCode=SS,PW,VE
  PS-Simulink Converter1 : nesl_utility/PS-Simulink Converter  PhysicalDomain=network_engine_domain  SubClassName=ps_output  LeftPortType=input  RightPortType=output  PseudoPeriodic=off  Frequencies=[]  VectorFormat=1-D array  Unit=V  AffineConversion=off
      settings: SourceProductBaseCode=SS,PW,VE
  PS-Simulink Converter2 : nesl_utility/PS-Simulink Converter  PhysicalDomain=network_engine_domain  SubClassName=ps_output  LeftPortType=input  RightPortType=output  PseudoPeriodic=off  Frequencies=[]  VectorFormat=1-D array  Unit=V  AffineConversion=off
      settings: SourceProductBaseCode=SS,PW,VE
  Voltage Sensor1 : fl_lib/Electrical/Electrical Sensors/Voltage Sensor
      settings: SourceProductBaseCode=PW,SS,VE
  Voltage Sensor2 : fl_lib/Electrical/Electrical Sensors/Voltage Sensor
      settings: SourceProductBaseCode=PW,SS,VE
  Voltage Sensor3 : fl_lib/Electrical/Electrical Sensors/Voltage Sensor
      settings: SourceProductBaseCode=PW,SS,VE
  AV : PMIOPort  Side=Left
  BV : PMIOPort  Port=2  Side=Left
  CV : PMIOPort  Port=3  Side=Left
  GND : PMIOPort  Port=4  Side=Left
  OUT : Outport
  wires:
  PS-Simulink Converter/1 -> Mux4/3
  PS-Simulink Converter1/1 -> Mux4/1
  PS-Simulink Converter2/1 -> Mux4/2
  Mux4/1 -> OUT/1
  connections:
  Voltage Sensor3/RConn2 -- Voltage Sensor1/RConn2 -- Voltage Sensor2/RConn2 -- GND/RConn1
  PS-Simulink Converter1/LConn1 -- Voltage Sensor1/RConn1
  Voltage Sensor3/LConn1 -- CV/RConn1
  PS-Simulink Converter2/LConn1 -- Voltage Sensor2/RConn1
  Voltage Sensor1/LConn1 -- AV/RConn1
  PS-Simulink Converter/LConn1 -- Voltage Sensor3/RConn1
  Voltage Sensor2/LConn1 -- BV/RConn1

== system MotorControl_Bldc/Subsystem4/GATED/Subsystem3 ==
  Mux4 : Mux  Inputs=3
  PS-Simulink Converter : nesl_utility/PS-Simulink Converter  PhysicalDomain=network_engine_domain  SubClassName=ps_output  LeftPortType=input  RightPortType=output  PseudoPeriodic=off  Frequencies=[]  VectorFormat=inherit  Unit=inherit  AffineConversion=off
      settings: SourceProductBaseCode=SS,PW,VE
  PS-Simulink Converter1 : nesl_utility/PS-Simulink Converter  PhysicalDomain=network_engine_domain  SubClassName=ps_output  LeftPortType=input  RightPortType=output  PseudoPeriodic=off  Frequencies=[]  VectorFormat=1-D array  Unit=V  AffineConversion=off
      settings: SourceProductBaseCode=SS,PW,VE
  PS-Simulink Converter2 : nesl_utility/PS-Simulink Converter  PhysicalDomain=network_engine_domain  SubClassName=ps_output  LeftPortType=input  RightPortType=output  PseudoPeriodic=off  Frequencies=[]  VectorFormat=1-D array  Unit=V  AffineConversion=off
      settings: SourceProductBaseCode=SS,PW,VE
  Voltage Sensor1 : fl_lib/Electrical/Electrical Sensors/Voltage Sensor
      settings: SourceProductBaseCode=PW,SS,VE
  Voltage Sensor2 : fl_lib/Electrical/Electrical Sensors/Voltage Sensor
      settings: SourceProductBaseCode=PW,SS,VE
  Voltage Sensor3 : fl_lib/Electrical/Electrical Sensors/Voltage Sensor
      settings: SourceProductBaseCode=PW,SS,VE
  AV : PMIOPort  Side=Left
  BV : PMIOPort  Port=2  Side=Left
  CV : PMIOPort  Port=3  Side=Left
  GND : PMIOPort  Port=4  Side=Left
  OUT : Outport
  wires:
  PS-Simulink Converter/1 -> Mux4/3
  PS-Simulink Converter1/1 -> Mux4/1
  PS-Simulink Converter2/1 -> Mux4/2
  Mux4/1 -> OUT/1
  connections:
  Voltage Sensor3/RConn2 -- Voltage Sensor1/RConn2 -- Voltage Sensor2/RConn2 -- GND/RConn1
  PS-Simulink Converter1/LConn1 -- Voltage Sensor1/RConn1
  Voltage Sensor3/LConn1 -- CV/RConn1
  PS-Simulink Converter2/LConn1 -- Voltage Sensor2/RConn1
  Voltage Sensor1/LConn1 -- AV/RConn1
  PS-Simulink Converter/LConn1 -- Voltage Sensor3/RConn1
  Voltage Sensor2/LConn1 -- BV/RConn1

== matlab function MotorControl_Bldc/XYZ ==
  data: Ualpha input; X output; Ubeta input; Ud input; Ts input; Y output; Z output
function [X,Y,Z] = fcn(Ualpha,Ubeta,Ud,Ts)
    X = sqrt(3)*Ubeta*Ts/Ud;
    Y = (3/2*Ualpha+sqrt(3)/2*Ubeta)*Ts/Ud;
    Z = (-3/2*Ualpha+sqrt(3)/2*Ubeta)*Ts/Ud;
end

== matlab function MotorControl_Bldc/Sector ==
  data: Ualpha input; y output; Ubeta input
function y = fcn(Ualpha,Ubeta)
y=1;
if Ualpha>=0&&Ubeta>=0&&Ualpha/Ubeta<=sqrt(3)
    y=1;
end
if Ubeta>=0&&Ubeta/abs(Ualpha)>=sqrt(3)
    y=2;
end
if Ualpha<=0&&Ubeta>=0&&-Ubeta/Ualpha<=sqrt(3)
    y=3;
end
if Ualpha<=0&&Ubeta<=0&&Ubeta/Ualpha<=sqrt(3)
    y=4;
end
if Ubeta<=0&&-Ubeta/abs(Ualpha)>=sqrt(3)
    y=5;
end
if Ualpha>=0&&Ubeta<=0&&-Ubeta/Ualpha<=sqrt(3)
    y=6;
end
end

== matlab function MotorControl_Bldc/TxTy ==
  data: N input; Tx output; X input; Y input; Z input; Ts input; Ty output; T0 output
function [Tx,Ty , T0] = fcn(N,X,Y,Z,Ts)
    switch N
        case 1
            Tx = -Z; Ty = X;
        case 2
            Tx = Z; Ty = Y;
        case 3
            Tx = X; Ty = -Y;
        case 4
            Tx = -X; Ty = Z;
        case 5
            Tx = -Y; Ty = -Z;
        case 6
            Tx = Y; Ty = -X;
        otherwise
            Tx = 0; Ty = 0;
    end
    if((Tx+Ty)>Ts)
        sum=Tx+Ty;
        k1=Tx/sum*Ts;
        k2=Ty/sum*Ts;
        Tx=k1;
        Ty=k2;
    end  
    T0=Ts-Tx-Ty;
end

== matlab function MotorControl_Bldc/TxTy1 ==
  data: N input; Ta output; T1 input; T2 input; T0 input; Ts input; Tb output; Tc output
function [Ta , Tb , Tc] = fcn(N,T1,T2,T0,Ts)
    switch N
        case 1
		    Ta = (T1 + T2 + T0/2);
			Tb = (T2 + T0/2);
			Tc = T0/2;
        case 2
			Ta = 1-(T1 +  T0/2);
			Tb = T1 + T2 + T0/2;
			Tc = T0/2;
        case 3
			Ta = T0/2;
			Tb = T1 + T2 + T0/2;
			Tc = T2 + T0/2;
        case 4
			Ta = T0/2;
			Tb = 1-(T1+ T0/2);
			Tc = (T1 + T2 + T0/2);
        case 5
			Ta = T2 + T0/2;
			Tb = T0/2;
			Tc = T1 + T2 + T0/2;
        case 6
 			Ta = T1 + T2 + T0/2;
			Tb = T0/2;
			Tc = 1-(T1 + T0/2);
        otherwise
  			Ta = 0;
			Tb = 0;
			Tc = 0;
    end
end

== matlab function MotorControl_Bldc/Sector3 ==
  data: Vd input; Vq input; Ud input; sintheta input; Ta output; costheta input; Tb output; Tc output
function [Ta , Tb , Tc] = fcn(Vd ,Vq , Ud,  sintheta ,costheta )
    sqrt3=sqrt(3);
    %%反park
    Ualpha=Vd*costheta-Vq*sintheta;
    Ubeta=Vd*sintheta+Vq*costheta;

    %%扇区判断dUq
    N=1;
    if (Ualpha>=0)&&(Ubeta>=0)&&(Ualpha/Ubeta<=sqrt3)
        N=1;
    end
    if (Ubeta>=0)&&(Ubeta/abs(Ualpha)>=sqrt3)
        N=2;
    end
    if (Ualpha<=0)&&(Ubeta>=0)&&(-Ubeta/Ualpha<=sqrt3)
        N=3;
    end
    if (Ualpha<=0)&&(Ubeta<=0)&&(Ubeta/Ualpha<=sqrt3)
        N=4;
    end
    if (Ubeta<=0)&&(-Ubeta/abs(Ualpha)>=sqrt3)
        N=5;
    end
    if (Ualpha>=0)&&(Ubeta<=0)&&(-Ubeta/Ualpha<=sqrt3)
        N=6;
    end
    
    
    %%中间量XYZ
    X = sqrt(3)*Ubeta*1/Ud;
    Y = (3/2*Ualpha+sqrt(3)/2*Ubeta)*1/Ud;
    Z = (-3/2*Ualpha+sqrt(3)/2*Ubeta)*1/Ud;
    
    %Tx ， Ty
    switch N
        case 1
            T1 = -Z; T2 = X;
        case 2
            T1 = Z; T2 = Y;
        case 3
            T1 = X; T2 = -Y;
        case 4
            T1 = -X; T2 = Z;
        case 5
            T1 = -Y; T2 = -Z;
        case 6
            T1 = Y; T2 = -X;
        otherwise
            T1 = 0; T2 = 0;
    end
    if((T1+T2)>1)
        sum=T1+T2;
        k1=T1/sum*1;
        k2=T2/sum*1;
        T1=k1;
        T2=k2;
    end  
    T0=1-T1-T2;
    
    %%Ta , Tb , Tc 
    switch N
        case 1
    	    Ta = (T1 + T2 + T0/2);
    		Tb = (T2 + T0/2);
    		Tc = T0/2;
        case 2
    		Ta = 1-(T1 +  T0/2);
    		Tb = T1 + T2 + T0/2;
    		Tc = T0/2;
        case 3
    		Ta = T0/2;
    		Tb = T1 + T2 + T0/2;
    		Tc = T2 + T0/2;
        case 4
    		Ta = T0/2;
    		Tb = 1-(T1+ T0/2);
    		Tc = (T1 + T2 + T0/2);
        case 5
    		Ta = T2 + T0/2;
    		Tb = T0/2;
    		Tc = T1 + T2 + T0/2;
        case 6
    		Ta = T1 + T2 + T0/2;
    		Tb = T0/2;
    		Tc = 1-(T1 + T0/2);
        otherwise
    		Ta = 0;
    		Tb = 0;
    		Tc = 0;
    end
end
